simulink library "DCCA_lib"  (Simulink 7.5)
settings: Solver=ode45  StartTime=0.0  StopTime=10.0  RelTol=1e-3
values from neighbouring files (symbols this model uses):
  p1_DCCA_DcDcTempThrsh_degC = Simulink.Parameter    [DCCA_par.m]
  p1_DCCA_DcDcVoltSetp_V = Simulink.Parameter    [DCCA_par.m]
  p_DCCA_TiDlyDcDcEnaP_s = Simulink.Parameter    [DCCA_par.m]
undefined symbols (not defined in the file or in its folder): DCDCAStsTyp, DCDCStsTyp
libraries: BaseOperationLib_Browser x12, PES_CZ_FAW x1, simulink x1
settings Model: Creator=wuaibin  LastModifiedBy=wuaibin

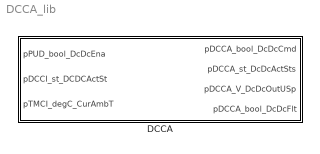
== system DCCA_lib ==
  DCCA : Subsystem  TreatAsAtomicUnit=on

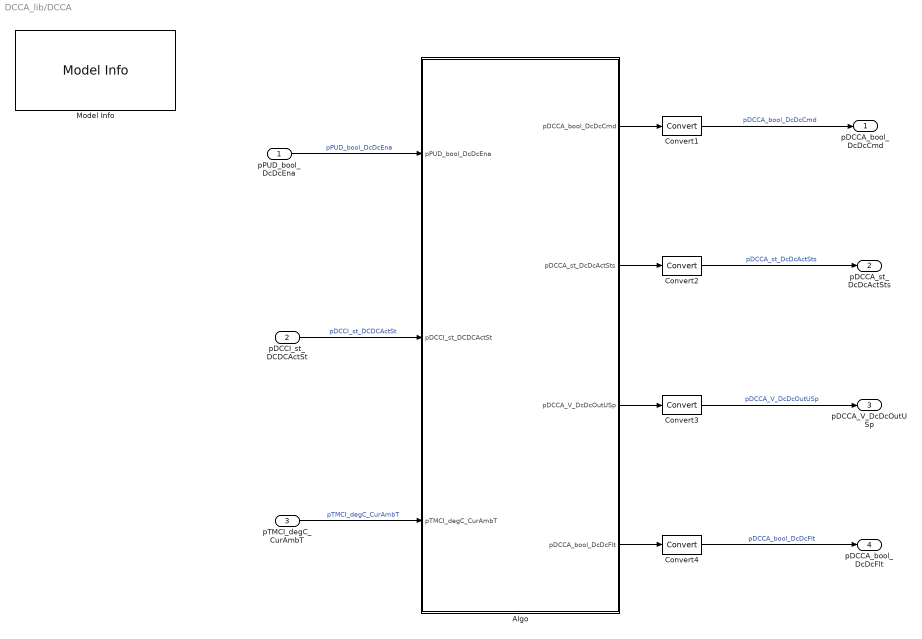
== system DCCA_lib/DCCA ==
  pPUD_bool_DcDcEna : Inport  OutDataType=fixdt(1, 16)  OutScaling=2^0
  pDCCI_st_DCDCActSt : Inport  Port=2  OutDataType=fixdt(1, 16)  OutScaling=2^0
  pTMCI_degC_CurAmbT : Inport  Port=3  OutDataType=fixdt(1, 16)  OutScaling=2^0
  Algo : Subsystem
  Convert{1..4} (4 alike) : DataTypeConversion  OutDataType=fixdt(1, 16)  OutScaling=2^0
  Model Info : simulink/Model-Wide Utilities/Model Info  SystemSampleTime=-1  InitialBlockCM=None  BlockCM=None  Frame=on  DisplayStringWithTags=Model Info\nCreated: %<Created>\nCreator: zhangqiang  HorizontalTextAlignment=Center  LeftAlignmentValue=0.5  SourceBlockDiagram=HQEV_HCU  TagMaxNumber=20
  pDCCA_bool_DcDcCmd : Outport  OutDataType=fixdt(1, 16)  OutScaling=2^0
  pDCCA_st_DcDcActSts : Outport  Port=2  OutDataType=fixdt(1, 16)  OutScaling=2^0
  pDCCA_V_DcDcOutUSp : Outport  Port=3  OutDataType=fixdt(1, 16)  OutScaling=2^0
  pDCCA_bool_DcDcFlt : Outport  Port=4  OutDataType=fixdt(1, 16)  OutScaling=2^0
  wires:
  Algo/4(pDCCA_bool_DcDcFlt) -> Convert4/1
  Algo/3(pDCCA_V_DcDcOutUSp) -> Convert3/1
  Algo/2(pDCCA_st_DcDcActSts) -> Convert2/1
  Algo/1(pDCCA_bool_DcDcCmd) -> Convert1/1
  pTMCI_degC_CurAmbT/1 -> Algo/3(pTMCI_degC_CurAmbT)  "pTMCI_degC_CurAmbT"
  pDCCI_st_DCDCActSt/1 -> Algo/2(pDCCI_st_DCDCActSt)  "pDCCI_st_DCDCActSt"
  pPUD_bool_DcDcEna/1 -> Algo/1(pPUD_bool_DcDcEna)  "pPUD_bool_DcDcEna"
  Convert4/1 -> pDCCA_bool_DcDcFlt/1  "pDCCA_bool_DcDcFlt"
  Convert3/1 -> pDCCA_V_DcDcOutUSp/1  "pDCCA_V_DcDcOutUSp"
  Convert2/1 -> pDCCA_st_DcDcActSts/1  "pDCCA_st_DcDcActSts"
  Convert1/1 -> pDCCA_bool_DcDcCmd/1  "pDCCA_bool_DcDcCmd"

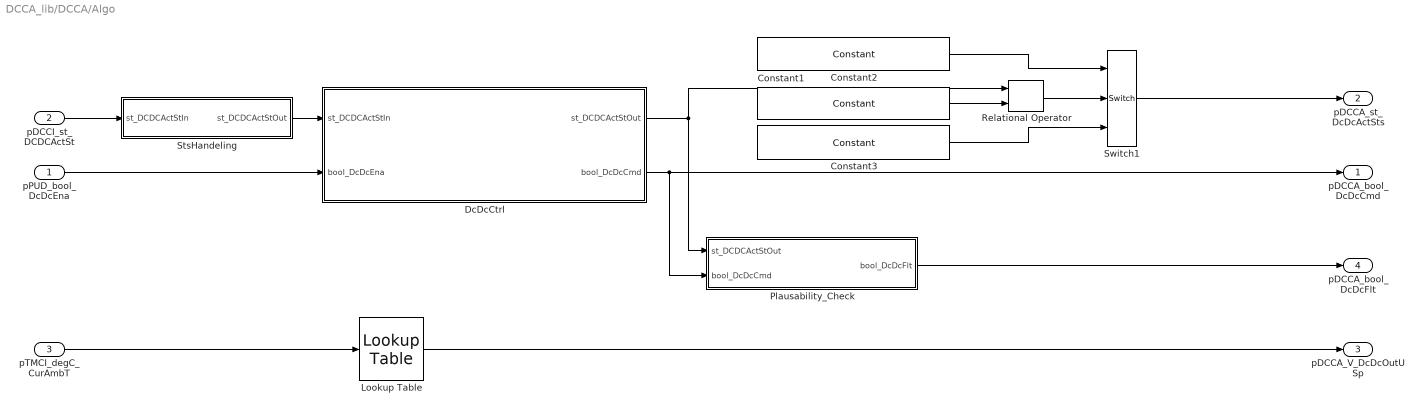
== system DCCA_lib/DCCA/Algo ==
  pPUD_bool_DcDcEna : Inport  OutDataType=fixdt(1, 16)  OutScaling=2^0
  pDCCI_st_DCDCActSt : Inport  Port=2  OutDataType=fixdt(1, 16)  OutScaling=2^0
  pTMCI_degC_CurAmbT : Inport  Port=3  OutDataType=fixdt(1, 16)  OutScaling=2^0
  Constant1 : BaseOperationLib_Browser/Sources&Sinks/Constant  Value=uint8(DCDCStsTyp.DCDC_ENA)  OutMin=[]  OutMax=[]  OutDataType=Enum: DCDCStsTyp  ConRadixGroup=Best Precision: Vector-wise  OutScaling=[]  OutDataTypeStr=Inherit: Inherit from 'Constant value'
  Constant2 : BaseOperationLib_Browser/Sources&Sinks/Constant  Value=uint8(DCDCAStsTyp.DST_Working)  OutMin=[]  OutMax=[]  OutDataType=Enum: DCDCAStsTyp  ConRadixGroup=Best Precision: Vector-wise  OutScaling=[]  OutDataTypeStr=Inherit: Inherit from 'Constant value'
  Constant3 : BaseOperationLib_Browser/Sources&Sinks/Constant  Value=uint8(DCDCAStsTyp.DST_ShutDown)  OutMin=[]  OutMax=[]  OutDataType=Enum: DCDCAStsTyp  ConRadixGroup=Best Precision: Vector-wise  OutScaling=[]  OutDataTypeStr=Inherit: Inherit from 'Constant value'
  DcDcCtrl : Stateflow chart  TreatAsAtomicUnit=on
  Lookup Table : BaseOperationLib_Browser/Lookup Tables Changed/Lookup Table  InputValues=p1_DCCA_DcDcTempThrsh_degC  Table=p1_DCCA_DcDcVoltSetp_V  LookUpMeth=Interpolation-Use End Values  OutMin=[]  OutMax=[]  OutDataType=fixdt(1, 16)  OutScaling=2^0  OutDataTypeStr=Inherit: Inherit via back propagation  SaturateOnIntegerOverflow=on
      settings: AttributesFormatString=X:%<InputValues>\nTAB:%<Table>
  Plausability_Check : Subsystem
  Relational Operator : BaseOperationLib_Browser/Logic Operations Changed/Relational Operator  Operator===  InputSameDT=on  LogicOutDataTypeMode=Specify via dialog  LogicDataType=PDT_Bool  OutDataTypeStr=PDT_Bool
  StsHandeling : Subsystem
  Switch1 : BaseOperationLib_Browser/Signal Routing Changed/Switch  Criteria=u2 ~= 0  Threshold=1  InputSameDT=on  OutMin=[]  OutMax=[]  OutDataType=fixdt(1,16,0)  OutScaling=[]  SaturateOnIntegerOverflow=on
  pDCCA_bool_DcDcCmd : Outport  OutDataType=fixdt(1, 16)  OutScaling=2^0
  pDCCA_st_DcDcActSts : Outport  Port=2  OutDataType=fixdt(1, 16)  OutScaling=2^0
  pDCCA_V_DcDcOutUSp : Outport  Port=3  OutDataType=fixdt(1, 16)  OutScaling=2^0
  pDCCA_bool_DcDcFlt : Outport  Port=4  OutDataType=fixdt(1, 16)  OutScaling=2^0
  wires:
  Lookup Table/1 -> pDCCA_V_DcDcOutUSp/1
  StsHandeling/1(st_DCDCActStOut) -> DcDcCtrl/1(st_DCDCActStIn)
  Constant3/1 -> Switch1/3
  Switch1/1 -> pDCCA_st_DcDcActSts/1
  Constant2/1 -> Switch1/1
  Relational Operator/1 -> Switch1/2
  Constant1/1 -> Relational Operator/2
  pTMCI_degC_CurAmbT/1 -> Lookup Table/1
  pPUD_bool_DcDcEna/1 -> DcDcCtrl/2(bool_DcDcEna)
  DcDcCtrl/2(bool_DcDcCmd) -> pDCCA_bool_DcDcCmd/1, Plausability_Check/2(bool_DcDcCmd)
  pDCCI_st_DCDCActSt/1 -> StsHandeling/1(st_DCDCActStIn)
  DcDcCtrl/1(st_DCDCActStOut) -> Relational Operator/1, Plausability_Check/1(st_DCDCActStOut)
  Plausability_Check/1(bool_DcDcFlt) -> pDCCA_bool_DcDcFlt/1

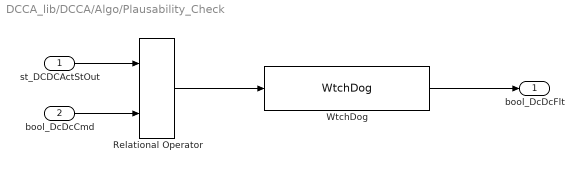
== system DCCA_lib/DCCA/Algo/Plausability_Check ==
  st_DCDCActStOut : Inport  OutDataType=fixdt(1, 16)  OutScaling=2^0
  bool_DcDcCmd : Inport  Port=2  OutDataType=fixdt(1, 16)  OutScaling=2^0
  Relational Operator : BaseOperationLib_Browser/Logic Operations Changed/Relational Operator  Operator===  InputSameDT=on  LogicOutDataTypeMode=Specify via dialog  LogicDataType=PDT_Bool  OutDataTypeStr=PDT_Bool
  WtchDog : PES_CZ_FAW/Discontinuities/WtchDog  SystemSampleTime=-1  timeoutthres=[p_DCCA_TiDlyDcDcEnaP_s]
  bool_DcDcFlt : Outport  OutDataType=fixdt(1, 16)  OutScaling=2^0
  wires:
  st_DCDCActStOut/1 -> Relational Operator/1
  bool_DcDcCmd/1 -> Relational Operator/2
  Relational Operator/1 -> WtchDog/1
  WtchDog/1 -> bool_DcDcFlt/1

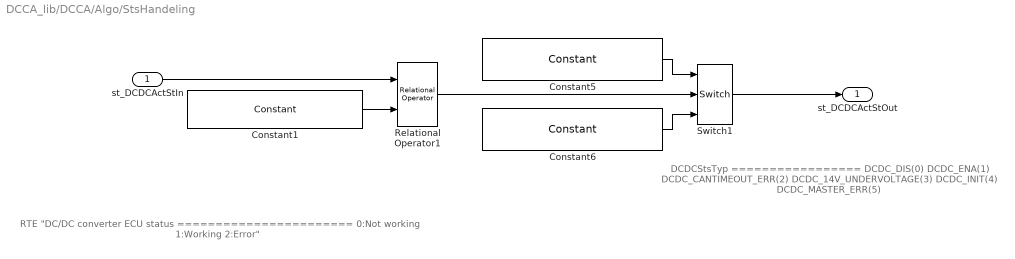
== system DCCA_lib/DCCA/Algo/StsHandeling ==
  note: DCDCStsTyp
      | =================
      |     DCDC_DIS(0)
      |     DCDC_ENA(1)
      |     DCDC_CANTIMEOUT_ERR(2)
      |     DCDC_14V_UNDERVOLTAGE(3)
      |     DCDC_INIT(4)
      |     DCDC_MASTER_ERR(5)
  note: RTE "DC/DC converter ECU status
      | =======================
      | 0:Not working
      | 1:Working
      | 2:Error"
  st_DCDCActStIn : Inport
  Constant1 : BaseOperationLib_Browser/Sources&Sinks/Constant  Value=uint8(DCDCStsTyp.DCDC_ENA)  OutMin=[]  OutMax=[]  OutDataType=fixdt(1, 16)  ConRadixGroup=Use specified scaling  OutScaling=2^0  OutDataTypeStr=Inherit: Inherit from 'Constant value'
  Constant5 : BaseOperationLib_Browser/Sources&Sinks/Constant  Value=uint8(DCDCStsTyp.DCDC_ENA)  OutMin=[]  OutMax=[]  OutDataType=fixdt(1, 16)  ConRadixGroup=Use specified scaling  OutScaling=2^0  OutDataTypeStr=Inherit: Inherit from 'Constant value'
  Constant6 : BaseOperationLib_Browser/Sources&Sinks/Constant  Value=uint8(DCDCStsTyp.DCDC_DIS)  OutMin=[]  OutMax=[]  OutDataType=fixdt(1, 16)  ConRadixGroup=Use specified scaling  OutScaling=2^0  OutDataTypeStr=Inherit: Inherit from 'Constant value'
  Relational Operator1 : BaseOperationLib_Browser/Logic Operations Changed/Relational Operator  Operator===  InputSameDT=on  LogicOutDataTypeMode=Specify via dialog  LogicDataType=PDT_Bool  OutDataTypeStr=PDT_Bool
  Switch1 : BaseOperationLib_Browser/Signal Routing Changed/Switch  Criteria=u2 ~= 0  Threshold=1  InputSameDT=on  OutMin=[]  OutMax=[]  OutDataType=fixdt(1,16,0)  OutScaling=[]  SaturateOnIntegerOverflow=on
  st_DCDCActStOut : Outport
  wires:
  st_DCDCActStIn/1 -> Relational Operator1/1
  Switch1/1 -> st_DCDCActStOut/1
  Constant1/1 -> Relational Operator1/2
  Relational Operator1/1 -> Switch1/2
  Constant5/1 -> Switch1/1
  Constant6/1 -> Switch1/3

== stateflow chart DCCA/Algo/DcDcCtrl ==
  state DCDCOff
    entry:
    bool_DcDcCmd = DCDCStsTyp.DCDC_DIS;
    settings: description=DCDC Converter is off (disabled).
    DCDCOff -> DCDCOff [order 1] : [st_DCDCActStIn == DCDCStsTyp.DCDC_DIS && ...
        | st_DCDCActStOut ~= DCDCStsTyp.DCDC_DIS]
        | {st_DCDCActStOut = DCDCStsTyp.DCDC_DIS;}
  state DCDCOn
    entry:
    bool_DcDcCmd = DCDCStsTyp.DCDC_ENA;
    settings: description=In this state, the DCDC Converter is turned on (enabled) and the output voltage setpoint is computed according the ambient temperature. A lookup table is used to translate the temperature into output voltage setpoint.
    DCDCOn -> DCDCOn [order 1] : [st_DCDCActStIn == DCDCStsTyp.DCDC_ENA && ...
        | st_DCDCActStOut ~= DCDCStsTyp.DCDC_ENA]
        | {st_DCDCActStOut = DCDCStsTyp.DCDC_ENA;}
  (default) -> DCDCOff : {st_DCDCActStOut = DCDCStsTyp.DCDC_DIS;}
  DCDCOn -> DCDCOff [order 1] : [!bool_DcDcEna]
    settings: description=Disable DCDC Converter if HV is not on or DCDC disable command is given by the BMS control.
  DCDCOff -> DCDCOn [order 1] : [bool_DcDcEna]
    settings: description=Enable DCDC Converter if HV is on and Energy Coordinator is not in error state and no DCDC disable command is given by the BMS control and the Converter is not in error state.
  data: st_DCDCActStOut output uint8; st_DCDCActStIn input double; bool_DcDcEna input boolean =0; bool_DcDcCmd output uint8 =DCDCStsTyp.DCDC_DIS
